simulink model "Projeto01"  (R2020a)
settings: Solver=VariableStepAuto  StartTime=0.0  StopTime=3  MaxStep=1e-3  RelTol=1e-3
settings Model: Creator=a1  LastModifiedBy=a1

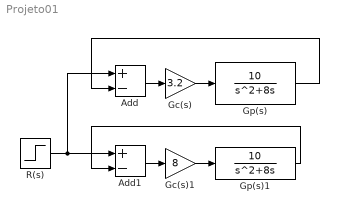
== system Projeto01 ==
  Add : Sum  Inputs=+-
  Add1 : Sum  Inputs=+-
  Gc(s) : Gain  Gain=3.2
  Gc(s)1 : Gain  Gain=8
  Gp(s) : TransferFcn  Numerator=[10]  Denominator=[1 8 0]
  Gp(s)1 : TransferFcn  Numerator=[10]  Denominator=[1 8 0]
  R(s) : Step  SampleTime=0
  wires:
  Gc(s)/1 -> Gp(s)/1
  Add/1 -> Gc(s)/1
  Gp(s)/1 -> Add/2
  Gp(s)1/1 -> Add1/2
  R(s)/1 -> Add/1, Add1/1
  Add1/1 -> Gc(s)1/1
  Gc(s)1/1 -> Gp(s)1/1
